simulink model "MPPTSolarChargeControllerModel"  (R2020b)
settings: Solver=VariableStepAuto  StartTime=0.0  StopTime=120  FixedStep=1
undefined symbols (not defined in the file): Ion, Lithium, sigbuilder_block
libraries: powerlib x7, simulink x2, powerlib_meascontrol x2, electricdrivelib x1, re_lib x1
settings Model: Creator=Rodney Tan  LastModifiedBy=kcroosonsa
settings SolverCC: AlgebraicLoopSolver=LineSearch
settings DataIOCC: ReturnWorkspaceOutputs=off
settings OptimizationCC: LifeSpan=inf
settings DebuggingCC: SFUnexpectedBacktrackingDiag=warning  SFNoUnconditionalDefaultTransitionDiag=warning  SFExecutionAtInitializationDiag=none  ArithmeticOperatorsInVariantConditions=warning
settings SFSimCC: SimUseLocalCustomCode=off  CustomCodeUndefinedFunction=UseInterfaceOnly
settings RTWCC: RTWUseLocalCustomCode=off  Toolchain=Microsoft Visual C++ 2019 v16.0 | nmake (64-bit Windows)  BuildConfiguration=Faster Runs
settings CodeAppCC: StateflowObjectComments=on
settings ConfigComp: CovMetricSettings=dw  CovSaveCumulativeToWorkspaceVar=on  CovSaveSingleToWorkspaceVar=on  CovExternalEMLEnable=off
settings SimscapeCC: SimscapeNormalizeSystem=off

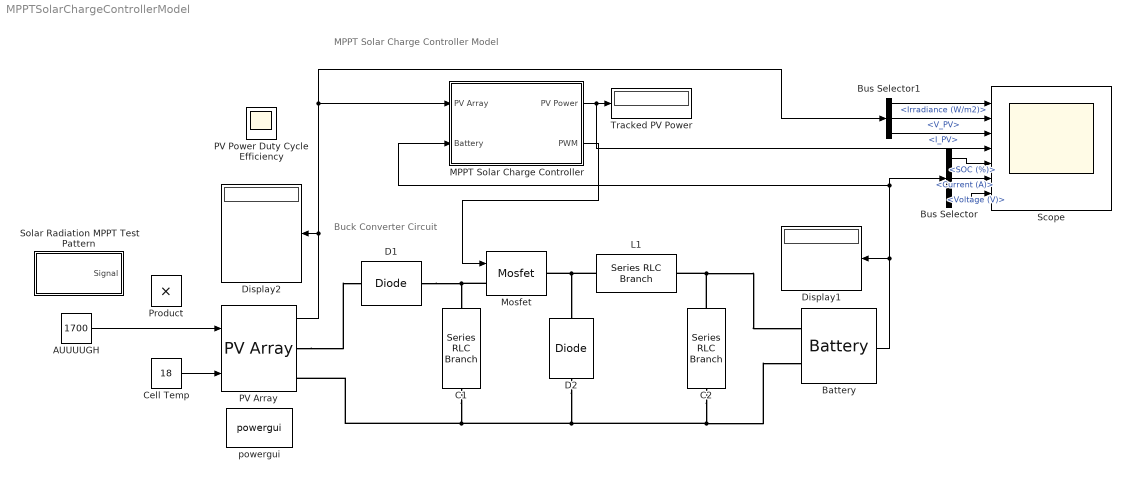
== system MPPTSolarChargeControllerModel ==
  note: MPPT Solar Charge Controller Model
  note: Buck Converter Circuit
  " C2" : powerlib/Elements/Series RLC Branch  LConnTagsString=__new0  RConnTagsString=__new0  BranchType=C  Resistance=0.1  Inductance=1e-3  SetiL0=off  InitialCurrent=0  Capacitance=1000e-6  Setx0=off  InitialVoltage=0  Measurements=None
  AUUUUGH : Constant  Value=1700
  Battery : electricdrivelib/Extra Sources/Battery  BatType=Lithium-Ion  ShowTempParam=off  ThermalPreset=no  ShowAgeParam=off  NomV=12.8  NomQ=100000000000  SOC=20  Batt_Tr=30  PresetModel=on  MaxQ=100000000000  MinV=9.6  FullV=14.899  Dis_rate=43478260869.5652  R=1.28e-12  Normal_OP=90434782608.6957  expZone="[13.828938906752      4913043478.2609]"  current=[6.5 13 32.5]  Units=Time  Tci=20  NomT=20  T2=-30  MaxQ2=4.8  FullV2=7.1  Normal_OP2=5.655  expZone2="[6.58           1]"  Rca=0.6  ti=2000  Dp=0  Neq0=0  Tsim=1e6  Ta1=25  Qeol=5.4*0.9  Reol=0.013333*1.2  Char_age=[2.3478, 3]  Dis_age=[2.3478, 10]  N1=1500  N2=10500  N3=1000  N4=1400  Ta2=45  N5=950
  Bus Selector : BusSelector  OutputSignals=SOC (%),Current (A),Voltage (V)
  Bus Selector1 : BusSelector  OutputSignals=Irradiance (W/m2),V_PV,I_PV
  C1 : powerlib/Elements/Series RLC Branch  LConnTagsString=__new0  RConnTagsString=__new0  BranchType=C  Resistance=0.1  Inductance=1e-3  SetiL0=off  InitialCurrent=0  Capacitance=1000e-6  Setx0=off  InitialVoltage=0  Measurements=None
  Cell Temp : Constant  Value=18
  D1 : powerlib/Power Electronics/Diode  Ron=0.001  Lon=0  Vf=0.8  IC=0  UseSnubber=0  Rs=inf  Cs=0  Measurements=off
  D2 : powerlib/Power Electronics/Diode  Ron=0.001  Lon=0  Vf=0.5  IC=0  UseSnubber=0  Rs=inf  Cs=0  Measurements=off
  Display1 : Display
  Display2 : Display
  L1 : powerlib/Elements/Series RLC Branch  LConnTagsString=__new0  RConnTagsString=__new0  BranchType=L  Resistance=1  Inductance=10e-3  SetiL0=off  InitialCurrent=0  Capacitance=1e-6  Setx0=off  InitialVoltage=0  Measurements=None
  MPPT Solar Charge Controller : Subsystem  mask(MPPT Solar Charge Controller Block){dD=1e-6, BattCV=12.8, Fsw=1000}
      mask prompts: dD "MPPT Duty Cycle (delta) Step Size"; BattCV "Battery Charging Constant Voltage (V)"; Fsw "PWM Switching frequency (Hz):"
      mask help:
      | MPPT Solar Charge Controller Block
      | Developed by Rodney Tan (PhD)
      | Version 1.00 Oct 2019
      |
      | This block perform solar photovoltaic Maximum Power Point Tracking based on Perturbation & Observation algorithm and charge lead acid battery using three stage charging algorithm.
      mask Help:
      | <b><u>Block Setting</u></b>
      | 
      | <b>MPPT Duty Cycle Step Size</b>
      | Specify the MPPT duty cycle (delta) step size. Default value is 1e-5.
      | 
      | <b>Battery Charging Constant Voltage (V)</b>
      | Specify the battery charging constant voltage for absorption stage.
      | 
      | <b>PWM Switching Frequency (Hz)</b>
      | Specify the PWM switching frequency in Hz.
      mask TypeOptions Fsw:
      | PWM Generator
      | (DC-DC)/Fsw
  Mosfet : powerlib/Power Electronics/Mosfet  Ron=0.02  Lon=0  Rd=0.01  Vfd=0  IC=0  Rs=1e5  Cs=inf  Measurements=off
  PV Array : re_lib/Solar/PV Array  Npar=1  Nser=1  PlotType=array @ 25 deg.C & specified irradiances  S_vec="[ 1000  800  600 400 200 ]"  Temp_C_vec="[ 45 25  ]"  ModuleName=User-defined  PlotWhenSelected=off  Pm=149.984  Ncell=60  Voc=21.6  Isc=9.72  Vm=17.2  Im=8.72  beta_Voc_pc=-0.36901  alpha_Isc_pc=0.086998  beta_Voc=-0.079706  alpha_Isc=0.0084562  IL=9.7783  I0=4.5547e-10  nI=0.59071  Rsh=33.058  Rs=0.19829  RobustModel=off  RobustCellTemperature=313.3991  BAL=off  Tc=1e-6  Tfilter=1e-5
  PV Power Duty Cycle Efficiency : Scope
      settings: Floating=on
  Product : Product
  Scope : Scope  NumInputPorts=7
  Solar Radiation MPPT Test Pattern : Subsystem  Tag=STV Subsys  LoadFcn=sigbuilder_block('load');  StartFcn=sigbuilder_block('start');  StopFcn=sigbuilder_block('stop');  ClipboardFcn=sigbuilder_block('clipboard');  mask(Sigbuilder block){tuvar=[0:10]}
      mask help: Simulink:masks:SigbuilderBlock_MD
      mask init:
      | if ~strcmp(get_param(bdroot(gcbh),'SimulationStatus'),'stopped') tuvar = sigbuilder_block('maskInit'); end
      settings: CopyFcn=sigbuilder_block('copy');  DeleteFcn=sigbuilder_block('delete');  ModelCloseFcn=sigbuilder_block('modelClose');  PreSaveFcn=sigbuilder_block('preSave');  PauseFcn=sigbuilder_block('pause');  ContinueFcn=sigbuilder_block('continue');  NameChangeFcn=sigbuilder_block('namechange');  OpenFcn=sigbuilder_block('open',[6 30 1428 771.75 ]);  CloseFcn=sigbuilder_block('close');
      mask Display: plot(0, 0, 100, 100,[2, 2, 32, 32, 2], [68, 8, 8, 68, 68],[32, 2], [38, 38], [32, 19, 2],[53, 60, 44], [32, 17, 17, 2],[16, 16, 31, 31]);txt = getActiveGroup(gcbh);text(2, 100, txt,'verticalAlignment', 'top');
  Tracked PV Power : Display
  powergui : powerlib/powergui  Priority=1  SimulationMode=Discrete  SampleTime=1e-4  frequency=60  Iterations=50  frequencyindice=0  Pbase=100e6  ErrMax=1e-4  UnitsV=kV  UnitsW=MW  buscounter=0  FunctionMessages=off  echomessages=off  EnableUseOfTLC=off  CurrentSourceSwitches=off  DisableSnubberDevices=off  DisableRonSwitches=off  DisableVfSwitches=off  DisplayEquations=off  AutomaticDiscreteSolvers=off  SolverType=Tustin/Backward Euler (TBE)  Interpol=off  ExternalGateDelay=off  methode=off  Ts=100  x0status=blocks  SPID=off  SwTol=0  HookPort=off  NonlinearTolerance=1e-4  nMaxIteration=100  ContinueOnMaxIteration=off  RestoreLinks=warning  ResistiveCurrentMeasurement=off  Frange=[0:2:500]  Ylog=off  Xlog=on  ShowGrid=off  save=off  variable=ZData  structure=0  ZoomFFT=off  StartTime=0.0  cycles=1  DisplayStyle=1  fundamental=60  FreqAxis=off  MaxFrequency=1000  frequencyindicesteady=1  RmsSteady=1  display=off
  wires:
  Cell Temp/1 -> PV Array/2
  PV Array/1 -> Bus Selector1/1, MPPT Solar Charge Controller/1(PV Array), Display2/1
  Battery/1 -> Bus Selector/1, MPPT Solar Charge Controller/2(Battery), Display1/1
  MPPT Solar Charge Controller/1(PV Power) -> Scope/4, Tracked PV Power/1
  MPPT Solar Charge Controller/2(PWM) -> Mosfet/1
  Bus Selector1/1 -> Scope/1  "<Irradiance (W/m2)>"
  Bus Selector1/2 -> Scope/2  "<V_PV>"
  Bus Selector/1 -> Scope/5  "<SOC (%)>"
  Bus Selector/2 -> Scope/6  "<Current (A)>"
  Bus Selector/3 -> Scope/7  "<Voltage (V)>"
  Bus Selector1/3 -> Scope/3  "<I_PV>"
  AUUUUGH/1 -> PV Array/1
  connections:
  " C2"/LConn1 -- Battery/LConn1 -- L1/RConn1
  Mosfet/LConn1 -- D1/RConn1 -- C1/LConn1
  " C2"/RConn1 -- Battery/LConn2 -- D2/LConn1 -- PV Array/RConn2 -- C1/RConn1
  L1/LConn1 -- D2/RConn1 -- Mosfet/RConn1
  PV Array/RConn1 -- D1/LConn1

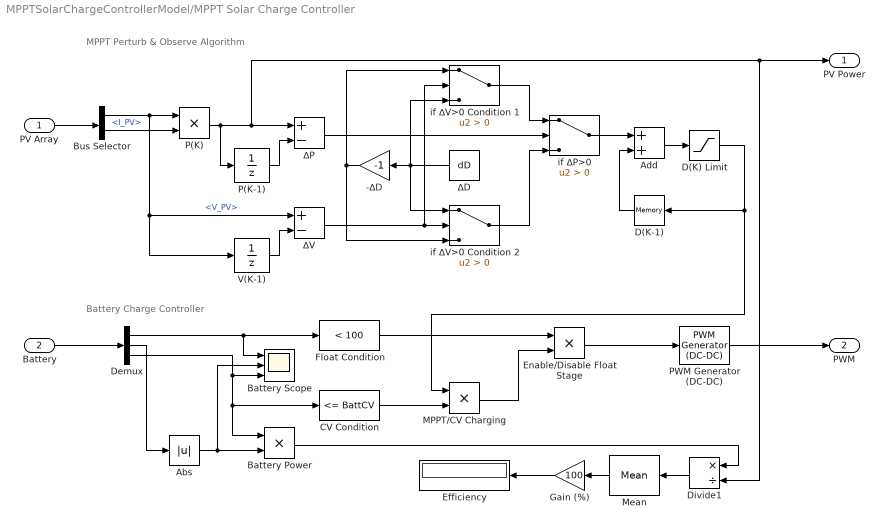
== system MPPTSolarChargeControllerModel/MPPT Solar Charge Controller ==
  note: Battery Charge Controller
  note: MPPT Perturb & Observe Algorithm
  PV Array : Inport
  Battery : Inport  Port=2
  -∆D : Gain  Gain=-1
  Abs : Abs
  Add : Sum
  Battery Power : Product
  Battery Scope : Scope  NumInputPorts=3
  Bus Selector : BusSelector  OutputSignals=V_PV,I_PV
  CV Condition : simulink/Logic and Bit Operations/Compare To Constant  relop=<=  const=BattCV  OutDataTypeStr=boolean
  D(K) Limit : Saturate  UpperLimit=0.6  LowerLimit=0.4
  D(K-1) : Memory  InitialCondition=0.5  InheritSampleTime=on  LinearizeMemory=on  LinearizeAsDelay=on
  Demux : Demux  Outputs=3
  Divide1 : Product  Inputs=*/
  Efficiency : Display
  Enable/Disable Float Stage : Product
  Float Condition : simulink/Logic and Bit Operations/Compare To Constant  relop=<  const=100  OutDataTypeStr=boolean
  Gain (%) : Gain  Gain=100
  MPPT/CV Charging : Product
  Mean : powerlib_meascontrol/Measurements/Mean  Freq=1  Vinit=0  Ts=0
  P(K) : Product
  P(K-1) : UnitDelay  SampleTime=-1  HasFrameUpgradeWarning=on
  PWM Generator (DC-DC) : powerlib_meascontrol/Pulse & Signal Generators/PWM Generator (DC-DC)  Fsw=Fsw  Ts=0
  V(K-1) : UnitDelay  SampleTime=-1  HasFrameUpgradeWarning=on
  if ∆P>0 : Switch  Criteria=u2 > Threshold
  if ∆V>0 Condition 1 : Switch  Criteria=u2 > Threshold
  if ∆V>0 Condition 2 : Switch  Criteria=u2 > Threshold
  ∆D : Constant  Value=dD
  ∆P : Sum  Inputs=+-
  ∆V : Sum  Inputs=+-
  PV Power : Outport  VectorParamsAs1DForOutWhenUnconnected=off
  PWM : Outport  Port=2  VectorParamsAs1DForOutWhenUnconnected=off
  wires:
  P(K)/1 -> ∆P/1, Divide1/2, PV Power/1, P(K-1)/1
  if ∆V>0 Condition 1/1 -> if ∆P>0/1
  ∆P/1 -> if ∆P>0/2
  P(K-1)/1 -> ∆P/2
  V(K-1)/1 -> ∆V/2
  ∆V/1 -> if ∆V>0 Condition 2/2, if ∆V>0 Condition 1/2
  Add/1 -> D(K) Limit/1
  if ∆V>0 Condition 2/1 -> if ∆P>0/3
  D(K-1)/1 -> Add/2
  ∆D/1 -> if ∆V>0 Condition 2/1, -∆D/1, if ∆V>0 Condition 1/3
  -∆D/1 -> if ∆V>0 Condition 2/3, if ∆V>0 Condition 1/1
  PWM Generator (DC-DC)/1 -> PWM/1
  Enable/Disable Float Stage/1 -> PWM Generator (DC-DC)/1
  Float Condition/1 -> Enable/Disable Float Stage/1
  CV Condition/1 -> MPPT/CV Charging/2
  Battery/1 -> Demux/1
  Demux/3 -> Battery Scope/3, CV Condition/1, Battery Power/1
  Demux/1 -> Float Condition/1, Battery Scope/1
  MPPT/CV Charging/1 -> Enable/Disable Float Stage/2
  Demux/2 -> Abs/1
  Divide1/1 -> Mean/1
  Mean/1 -> Gain (%)/1
  Abs/1 -> Battery Scope/2, Battery Power/2
  Bus Selector/2 -> P(K)/2  "<I_PV>"
  Battery Power/1 -> Divide1/1
  Bus Selector/1 -> ∆V/1, V(K-1)/1, P(K)/1  "<V_PV>"
  PV Array/1 -> Bus Selector/1
  if ∆P>0/1 -> Add/1
  D(K) Limit/1 -> D(K-1)/1, MPPT/CV Charging/1
  Gain (%)/1 -> Efficiency/1

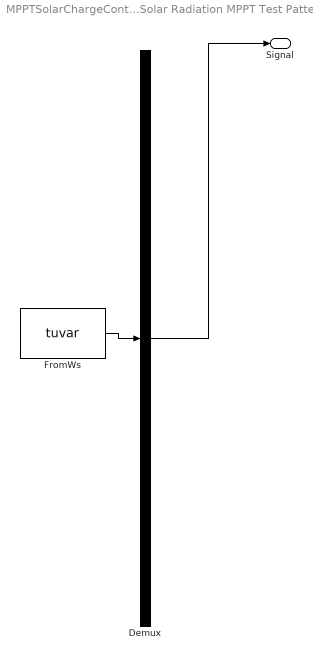
== system MPPTSolarChargeControllerModel/Solar Radiation MPPT Test Pattern ==
  Demux : Demux  Tag=STV Demux  Outputs=1
      settings: DisplayOption=none
  FromWs : FromWorkspace  Tag=STV FromWs  VariableName=tuvar
      SigBuilderData=|
      | common.afterFinalStr = 'Extrapolate'
      | common.sampleTime = 0
      | dataSet.timeRange = [0 86400]
      | dataSet.name = 'Test Pattern 1'
      | sbobj.Groups.Name = 'Test Pattern 1'
      | sbobj.Groups.Signals.Name = 'Signal'
      | sbobj.Groups.Signals.XData = [0 7200 7201 14400 14400 21600 21600 28800 28800 36000 36000 43200 43200 50400 50400 57600 57600 64800 64800 86400]
      | sbobj.Groups.Signals.YData = [100 100 200 200 300 300 400 400 500 500 600 600 700 700 638 638 520 520 354 100]
      | sbobj.Groups.TimeRange = [0 86400]
  Signal : Outport  Tag=STV Outport  VectorParamsAs1DForOutWhenUnconnected=off
  wires:
  FromWs/1 -> Demux/1
  Demux/1 -> Signal/1
